simulink model "Van_der_Pol"  (R2016b)
settings: Solver=VariableStepAuto  StartTime=0.0  StopTime=50  MaxStep=0.01  RelTol=1e-3
libraries: simulink x1
settings Model: Creator=BOUDOT  LastModifiedBy=BOUDOT

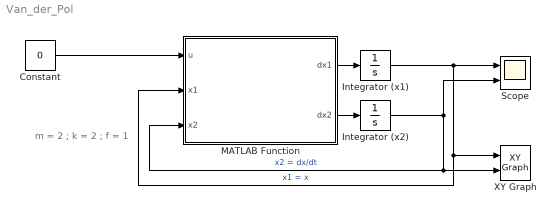
== system Van_der_Pol ==
  note: m = 2 ; k = 2 ; f = 1
  Constant : Constant  Value=0
  Integrator (x1) : Integrator  InitialCondition=1
  Integrator (x2) : Integrator  InitialCondition=0.4
  MATLAB Function : MATLAB Function  TreatAsAtomicUnit=on
  Scope : Scope  NumInputPorts=2
  XY Graph : simulink/Sinks/XY Graph  xmin=-5  xmax=5  ymin=-5  ymax=5  st=-1
  wires:
  MATLAB Function/1(dx1) -> Integrator (x1)/1
  MATLAB Function/2(dx2) -> Integrator (x2)/1
  Integrator (x2)/1 -> MATLAB Function/3(x2), XY Graph/2, Scope/2  "x2 = dx/dt"
  Integrator (x1)/1 -> Scope/1, XY Graph/1, MATLAB Function/2(x1)  "x1 = x"
  Constant/1 -> MATLAB Function/1(u)

== matlab function Van_der_Pol/MATLAB Function ==
  data: u input; dx1 output; x1 input; x2 input; dx2 output
function [dx1, dx2] = system(u, x1, x2)

e = 1;

dx1 = x2;
dx2 = -x1 - e*(x1^2-1)*x2 + u;
